simulink model "Demo_FrictionSensor_cs"  (Simulink 7.6)
settings: Solver=ode5  SolverMode=SingleTasking  StartTime=0.0  StopTime=12  FixedStep=1/200  RelTol=1e-3
PreLoadFcn:
  | check_NUTS_defined;
  | 
  | assignin('base',['model_closed_' bdroot],false);
InitFcn:
  | PreScanExperimentInitFcn(bdroot)
StopFcn:
  | PreScanExperimentStopFcn(bdroot)
undefined symbols (not defined in the file): DiscIntNeverNeededParam, warningInitialVelocity, x0, x_ini_VRML, y_ini_VRML, z_ini_VRML
libraries: simulink x40, PreScanSimulinkLibrary x15, simulink_extras x9, PreScanUsefulBlocks x3
(part 6 of 7)

== system Demo_FrictionSensor_cs/Audi_A8_1/PathFollower_Preview_1/LateralController/SteeringWheelAngle/FirstOrderDynamics ==
  In : Inport
  TimeConstant[s] : Inport  Port=2
  Reset : Inport  Port=3
  x0 : Inport  Port=4
  1|TimeConstant : Product  Inputs=*/  SaturateOnIntegerOverflow=on  InputSameDT=on  OutDataTypeStr=Inherit: Same as first input
  Discrete-Time Integrator : DiscreteIntegrator  ExternalReset=rising  InitialConditionSource=external  InitialCondition=x0  SampleTime=CSSampleTime  ICPrevOutput=DiscIntNeverNeededParam  ICPrevScaledInput=DiscIntNeverNeededParam
  IC : InitialCondition  Value=0
  Saturation : Saturate  UpperLimit=1e300  LowerLimit=0.001
  Sum : Sum  Inputs=-+|  SaturateOnIntegerOverflow=on  InputSameDT=on  OutDataTypeStr=Inherit: Same as first input
  Out : Outport
  wires:
  IC/1 -> Discrete-Time Integrator/3
  In/1 -> Sum/2
  x0/1 -> IC/1
  Reset/1 -> Discrete-Time Integrator/2
  1|TimeConstant/1 -> Discrete-Time Integrator/1
  Sum/1 -> 1|TimeConstant/1
  Saturation/1 -> 1|TimeConstant/2
  TimeConstant[s]/1 -> Saturation/1
  Discrete-Time Integrator/1 -> Out/1, Sum/1

== system Demo_FrictionSensor_cs/Audi_A8_1/PathFollower_Preview_1/LateralController/SteeringWheelAngle/Sat_Total ==
  In : Inport
  Sat_Limit : Inport  Port=2
  Gain1 : Gain  Gain=-1  SaturateOnIntegerOverflow=on  OutDataTypeStr=Inherit: Same as input  ParamDataTypeStr=Inherit: Same as input
  RelOp_UL : RelationalOperator
  RelOp_UL1 : RelationalOperator  Operator=<=
  Sum : Sum  Inputs=++|  SaturateOnIntegerOverflow=on
  Switch : Switch  Threshold=0.5  SaturateOnIntegerOverflow=on
  Switch1 : Switch  Threshold=0.5  SaturateOnIntegerOverflow=on
  Sat_Total : Outport
  Sat_Info : Outport  Port=2
  wires:
  Sat_Limit/1 -> Gain1/1, Switch/1, RelOp_UL/2
  RelOp_UL/1 -> Switch/2, Sum/2
  Switch/1 -> RelOp_UL1/1, Switch1/3
  Gain1/1 -> RelOp_UL1/2, Switch1/1
  RelOp_UL1/1 -> Switch1/2, Sum/1
  In/1 -> Switch/3, RelOp_UL/1
  Switch1/1 -> Sat_Total/1
  Sum/1 -> Sat_Info/1

== system Demo_FrictionSensor_cs/Audi_A8_1/PathFollower_Preview_1/LongitudinalController/If Desired Velocity ~= 0/PID Controller ==
  e : Inport
  Derivative Gain : Gain  Gain=D  SaturateOnIntegerOverflow=on  OutDataTypeStr=Inherit: Same as input  ParamDataTypeStr=Inherit: Same as input
  Discrete-Time Integrator : DiscreteIntegrator  gainval=1  SampleTime=CSSampleTime  ICPrevOutput=DiscIntNeverNeededParam  ICPrevScaledInput=DiscIntNeverNeededParam
  Filter : DiscreteIntegrator  gainval=1  SampleTime=CSSampleTime  ICPrevOutput=DiscIntNeverNeededParam  ICPrevScaledInput=DiscIntNeverNeededParam
  Integral Gain : Gain  Gain=I  SaturateOnIntegerOverflow=on  OutDataTypeStr=Inherit: Same as input  ParamDataTypeStr=Inherit: Same as input
  Proportional Gain : Gain  Gain=P  SaturateOnIntegerOverflow=on  OutDataTypeStr=Inherit: Same as input  ParamDataTypeStr=Inherit: Same as input
  Sum : Sum  Inputs=+++  SaturateOnIntegerOverflow=on  InputSameDT=on  OutDataTypeStr=Inherit: Same as first input
  Sum1 : Sum  Inputs=|+-  SaturateOnIntegerOverflow=on  InputSameDT=on  OutDataTypeStr=Inherit: Same as first input
  u : Outport  InitialOutput=0
  wires:
  Sum1/1 -> Filter/1, Sum/3
  Filter/1 -> Sum1/2
  Derivative Gain/1 -> Sum1/1
  Sum/1 -> u/1
  e/1 -> Integral Gain/1, Proportional Gain/1, Derivative Gain/1
  Discrete-Time Integrator/1 -> Sum/2
  Proportional Gain/1 -> Sum/1
  Integral Gain/1 -> Discrete-Time Integrator/1

== system Demo_FrictionSensor_cs/Audi_A8_1/PreScan_Contact_Sensor/Vehicle Local to World/state2FullState/Transformation_BODY2GLOBAL1 ==
  POSvector_BODY_[m] : Inport
  angles_BODYwrtGLOB_[rad] : Inport  Port=2
  Dot Product : DotProduct  InputSameDT=on  OutDataTypeStr=Inherit: Inherit via internal rule
  Dot Product1 : DotProduct  InputSameDT=on  OutDataTypeStr=Inherit: Inherit via internal rule
  Dot Product2 : DotProduct  InputSameDT=on  OutDataTypeStr=Inherit: Inherit via internal rule
  Fcn10 : Fcn  Expr=cos(u(1))*sin(u(2))*sin(u(3))-sin(u(1))*cos(u(3))
  Fcn11 : Fcn  Expr=cos(u(1))*sin(u(2))*cos(u(3))+sin(u(1))*sin(u(3))
  Fcn12 : Fcn  Expr=sin(u(1))*cos(u(2))
  Fcn13 : Fcn  Expr=sin(u(1))*sin(u(2))*sin(u(3))+cos(u(1))*cos(u(3))
  Fcn14 : Fcn  Expr=sin(u(1))*sin(u(2))*cos(u(3))-cos(u(1))*sin(u(3))
  Fcn15 : Fcn  Expr=-sin(u(2))
  Fcn16 : Fcn  Expr=cos(u(2))*sin(u(3))
  Fcn17 : Fcn  Expr=cos(u(2))*cos(u(3))
  Fcn9 : Fcn  Expr=cos(u(1))*cos(u(2))
  Mux1 : Mux  Inputs=9
  Mux3 : Mux  Inputs=3
  Selector : Selector  InputPortWidth=9  IndexOptions=Index vector (dialog)  Indices=[1 2 3]  OutputSizes=1
  Selector1 : Selector  InputPortWidth=9  IndexOptions=Index vector (dialog)  Indices=[4 5 6]  OutputSizes=1
  Selector2 : Selector  InputPortWidth=9  IndexOptions=Index vector (dialog)  Indices=[7 8 9]  OutputSizes=1
  rot_xyz 2 rot_zyx : Selector  InputPortWidth=3  IndexOptions=Index vector (dialog)  Indices=[3 2 1]  OutputSizes=1
  POSvector_GLOBAL_[m] : Outport
  wires:
  angles_BODYwrtGLOB_[rad]/1 -> rot_xyz 2 rot_zyx/1
  Mux3/1 -> POSvector_GLOBAL_[m]/1
  rot_xyz 2 rot_zyx/1 -> Fcn17/1, Fcn16/1, Fcn15/1, Fcn14/1, Fcn13/1, Fcn12/1, Fcn11/1, Fcn10/1, Fcn9/1
  Dot Product1/1 -> Mux3/2
  Dot Product2/1 -> Mux3/3
  Selector2/1 -> Dot Product2/2
  Selector1/1 -> Dot Product1/2
  Dot Product/1 -> Mux3/1
  POSvector_BODY_[m]/1 -> Dot Product/1, Dot Product1/1, Dot Product2/1
  Selector/1 -> Dot Product/2
  Mux1/1 -> Selector2/1, Selector1/1, Selector/1  "RotationMatrix"
  Fcn17/1 -> Mux1/9
  Fcn16/1 -> Mux1/8
  Fcn15/1 -> Mux1/7
  Fcn14/1 -> Mux1/6
  Fcn13/1 -> Mux1/5
  Fcn12/1 -> Mux1/4
  Fcn11/1 -> Mux1/3
  Fcn10/1 -> Mux1/2
  Fcn9/1 -> Mux1/1

== system Demo_FrictionSensor_cs/Audi_A8_1/PreScan_Contact_Sensor/Vehicle Local to World/state2FullState/limit roll ==
  RPY : Inport
  Demux : Demux  Outputs=3
  Mux1 : Mux  Inputs=3
  Substitute 90 & 270 deg (and its plurals) : Subsystem
  RPYcor : Outport
  wires:
  Demux/1 -> Substitute 90 & 270 deg (and its plurals)/1(Angle [rad])
  Demux/2 -> Mux1/2
  Demux/3 -> Mux1/3
  RPY/1 -> Demux/1
  Mux1/1 -> RPYcor/1
  Substitute 90 & 270 deg (and its plurals)/1(Subst Angle [rad]) -> Mux1/1

== system Demo_FrictionSensor_cs/Audi_A8_1/PreScan_Contact_Sensor/Wheels Local to World/conv_RotWheelFL/RotMat2AxisAngle ==
  RotMat_Visu : Inport
  Data Type Conversion : DataTypeConversion
  Divide : Product  Inputs=*/
  Gain : Gain  Gain=2
  Mux : Mux  Inputs=3
  Mux1 : Mux  Inputs=2
  Saturation1 : Saturate  UpperLimit=3-0.001  LowerLimit=-1+0.001
  Trigonometric Function : Trigonometry
  U1 : Fcn  Expr=u[6]-u[8]
  U2 : Fcn  Expr=u[7]-u[3]
  U3 : Fcn  Expr=u[2]-u[4]
  U_Phi : Fcn  Expr=u[1]+u[5]+u[9]
  U_Phi1 : Fcn  Expr=acos((u(1)-1)/2)
  U_Phi2 : Fcn  Expr=acos((u(1)-1)/2)
  Angles_Visu : Outport
  wires:
  Data Type Conversion/1 -> Mux1/2
  RotMat_Visu/1 -> U1/1, U2/1, U3/1, U_Phi/1
  Trigonometric Function/1 -> Gain/1
  U1/1 -> Mux/1
  U2/1 -> Mux/2
  U3/1 -> Mux/3
  Mux/1 -> Divide/1
  Gain/1 -> Divide/2
  Mux1/1 -> Angles_Visu/1
  Divide/1 -> Mux1/1
  U_Phi/1 -> U_Phi1/1, Saturation1/1
  U_Phi1/1 -> Data Type Conversion/1
  Saturation1/1 -> U_Phi2/1
  U_Phi2/1 -> Trigonometric Function/1

== system Demo_FrictionSensor_cs/Audi_A8_1/PreScan_Contact_Sensor/Wheels Local to World/conv_RotWheelFR/RotMat2AxisAngle ==
  RotMat_Visu : Inport
  Data Type Conversion : DataTypeConversion
  Divide : Product  Inputs=*/
  Gain : Gain  Gain=2
  Mux : Mux  Inputs=3
  Mux1 : Mux  Inputs=2
  Saturation1 : Saturate  UpperLimit=3-0.001  LowerLimit=-1+0.001
  Trigonometric Function : Trigonometry
  U1 : Fcn  Expr=u[6]-u[8]
  U2 : Fcn  Expr=u[7]-u[3]
  U3 : Fcn  Expr=u[2]-u[4]
  U_Phi : Fcn  Expr=u[1]+u[5]+u[9]
  U_Phi1 : Fcn  Expr=acos((u(1)-1)/2)
  U_Phi2 : Fcn  Expr=acos((u(1)-1)/2)
  Angles_Visu : Outport
  wires:
  U_Phi2/1 -> Trigonometric Function/1
  Saturation1/1 -> U_Phi2/1
  U_Phi1/1 -> Data Type Conversion/1
  U_Phi/1 -> Saturation1/1, U_Phi1/1
  Divide/1 -> Mux1/1
  Mux1/1 -> Angles_Visu/1
  Gain/1 -> Divide/2
  Mux/1 -> Divide/1
  U3/1 -> Mux/3
  U2/1 -> Mux/2
  U1/1 -> Mux/1
  Trigonometric Function/1 -> Gain/1
  RotMat_Visu/1 -> U_Phi/1, U3/1, U2/1, U1/1
  Data Type Conversion/1 -> Mux1/2

== system Demo_FrictionSensor_cs/Audi_A8_1/PreScan_Contact_Sensor/Wheels Local to World/conv_RotWheelRL/RotMat2AxisAngle ==
  RotMat_Visu : Inport
  Data Type Conversion : DataTypeConversion
  Divide : Product  Inputs=*/
  Gain : Gain  Gain=2
  Mux : Mux  Inputs=3
  Mux1 : Mux  Inputs=2
  Saturation1 : Saturate  UpperLimit=3-0.001  LowerLimit=-1+0.001
  Trigonometric Function : Trigonometry
  U1 : Fcn  Expr=u[6]-u[8]
  U2 : Fcn  Expr=u[7]-u[3]
  U3 : Fcn  Expr=u[2]-u[4]
  U_Phi : Fcn  Expr=u[1]+u[5]+u[9]
  U_Phi1 : Fcn  Expr=acos((u(1)-1)/2)
  U_Phi2 : Fcn  Expr=acos((u(1)-1)/2)
  Angles_Visu : Outport
  wires:
  U_Phi2/1 -> Trigonometric Function/1
  Saturation1/1 -> U_Phi2/1
  U_Phi1/1 -> Data Type Conversion/1
  U_Phi/1 -> Saturation1/1, U_Phi1/1
  Divide/1 -> Mux1/1
  Mux1/1 -> Angles_Visu/1
  Gain/1 -> Divide/2
  Mux/1 -> Divide/1
  U3/1 -> Mux/3
  U2/1 -> Mux/2
  U1/1 -> Mux/1
  Trigonometric Function/1 -> Gain/1
  RotMat_Visu/1 -> U_Phi/1, U3/1, U2/1, U1/1
  Data Type Conversion/1 -> Mux1/2

== system Demo_FrictionSensor_cs/Audi_A8_1/PreScan_Contact_Sensor/Wheels Local to World/conv_RotWheelRR/RotMat2AxisAngle ==
  RotMat_Visu : Inport
  Data Type Conversion : DataTypeConversion
  Divide : Product  Inputs=*/
  Gain : Gain  Gain=2
  Mux : Mux  Inputs=3
  Mux1 : Mux  Inputs=2
  Saturation1 : Saturate  UpperLimit=3-0.001  LowerLimit=-1+0.001
  Trigonometric Function : Trigonometry
  U1 : Fcn  Expr=u[6]-u[8]
  U2 : Fcn  Expr=u[7]-u[3]
  U3 : Fcn  Expr=u[2]-u[4]
  U_Phi : Fcn  Expr=u[1]+u[5]+u[9]
  U_Phi1 : Fcn  Expr=acos((u(1)-1)/2)
  U_Phi2 : Fcn  Expr=acos((u(1)-1)/2)
  Angles_Visu : Outport
  wires:
  U_Phi2/1 -> Trigonometric Function/1
  Saturation1/1 -> U_Phi2/1
  U_Phi1/1 -> Data Type Conversion/1
  U_Phi/1 -> Saturation1/1, U_Phi1/1
  Divide/1 -> Mux1/1
  Mux1/1 -> Angles_Visu/1
  Gain/1 -> Divide/2
  Mux/1 -> Divide/1
  U3/1 -> Mux/3
  U2/1 -> Mux/2
  U1/1 -> Mux/1
  Trigonometric Function/1 -> Gain/1
  RotMat_Visu/1 -> U_Phi/1, U3/1, U2/1, U1/1
  Data Type Conversion/1 -> Mux1/2

== system Demo_FrictionSensor_cs/Audi_A8_1/PreScan_Contact_Sensor/Wheels Local to World/conv_TransWheelFL/pos_ini_Visu ==
  Constant : Constant  Value=x_ini_VRML
  Constant1 : Constant  Value=y_ini_VRML
  Constant2 : Constant  Value=z_ini_VRML
  Mux1 : Mux  Inputs=3
  pos_ini_Visu : Outport
  wires:
  Constant/1 -> Mux1/1
  Mux1/1 -> pos_ini_Visu/1
  Constant1/1 -> Mux1/2
  Constant2/1 -> Mux1/3

== system Demo_FrictionSensor_cs/Audi_A8_1/PreScan_Contact_Sensor/Wheels Local to World/conv_TransWheelFL/transISO2Visu ==
  transISO : Inport
  Demux : Demux  Outputs=3
  trans_x_Visu : Outport
  trans_y_Visu : Outport  Port=2
  trans_z_Visu : Outport  Port=3
  wires:
  Demux/2 -> trans_y_Visu/1  "rot_y"
  Demux/1 -> trans_x_Visu/1
  transISO/1 -> Demux/1
  Demux/3 -> trans_z_Visu/1

== system Demo_FrictionSensor_cs/Audi_A8_1/PreScan_Contact_Sensor/Wheels Local to World/conv_TransWheelFR/pos_ini_Visu ==
  Constant : Constant  Value=x_ini_VRML
  Constant1 : Constant  Value=y_ini_VRML
  Constant2 : Constant  Value=z_ini_VRML
  Mux1 : Mux  Inputs=3
  pos_ini_Visu : Outport
  wires:
  Constant2/1 -> Mux1/3
  Constant1/1 -> Mux1/2
  Mux1/1 -> pos_ini_Visu/1
  Constant/1 -> Mux1/1

== system Demo_FrictionSensor_cs/Audi_A8_1/PreScan_Contact_Sensor/Wheels Local to World/conv_TransWheelFR/transISO2Visu ==
  transISO : Inport
  Demux : Demux  Outputs=3
  trans_x_Visu : Outport
  trans_y_Visu : Outport  Port=2
  trans_z_Visu : Outport  Port=3
  wires:
  Demux/2 -> trans_y_Visu/1  "rot_y"
  Demux/1 -> trans_x_Visu/1
  transISO/1 -> Demux/1
  Demux/3 -> trans_z_Visu/1

== system Demo_FrictionSensor_cs/Audi_A8_1/PreScan_Contact_Sensor/Wheels Local to World/conv_TransWheelRL/pos_ini_Visu ==
  Constant : Constant  Value=x_ini_VRML
  Constant1 : Constant  Value=y_ini_VRML
  Constant2 : Constant  Value=z_ini_VRML
  Mux1 : Mux  Inputs=3
  pos_ini_Visu : Outport
  wires:
  Constant2/1 -> Mux1/3
  Constant1/1 -> Mux1/2
  Mux1/1 -> pos_ini_Visu/1
  Constant/1 -> Mux1/1

== system Demo_FrictionSensor_cs/Audi_A8_1/PreScan_Contact_Sensor/Wheels Local to World/conv_TransWheelRL/transISO2Visu ==
  transISO : Inport
  Demux : Demux  Outputs=3
  trans_x_Visu : Outport
  trans_y_Visu : Outport  Port=2
  trans_z_Visu : Outport  Port=3
  wires:
  Demux/2 -> trans_y_Visu/1  "rot_y"
  Demux/1 -> trans_x_Visu/1
  transISO/1 -> Demux/1
  Demux/3 -> trans_z_Visu/1

== system Demo_FrictionSensor_cs/Audi_A8_1/PreScan_Contact_Sensor/Wheels Local to World/conv_TransWheelRR/pos_ini_Visu ==
  Constant : Constant  Value=x_ini_VRML
  Constant1 : Constant  Value=y_ini_VRML
  Constant2 : Constant  Value=z_ini_VRML
  Mux1 : Mux  Inputs=3
  pos_ini_Visu : Outport
  wires:
  Constant2/1 -> Mux1/3
  Constant1/1 -> Mux1/2
  Mux1/1 -> pos_ini_Visu/1
  Constant/1 -> Mux1/1

== system Demo_FrictionSensor_cs/Audi_A8_1/PreScan_Contact_Sensor/Wheels Local to World/conv_TransWheelRR/transISO2Visu ==
  transISO : Inport
  Demux : Demux  Outputs=3
  trans_x_Visu : Outport
  trans_y_Visu : Outport  Port=2
  trans_z_Visu : Outport  Port=3
  wires:
  Demux/2 -> trans_y_Visu/1  "rot_y"
  Demux/1 -> trans_x_Visu/1
  transISO/1 -> Demux/1
  Demux/3 -> trans_z_Visu/1

== system Demo_FrictionSensor_cs/Audi_A8_1/Trajectories/Traj2State1/Traj2State2/MuxState ==
  x [m] : Inport
  y [m] : Inport  Port=2
  z [m] : Inport  Port=3
  dx [m/s] : Inport  Port=4
  dy [m/s] : Inport  Port=5
  dz [m/s] : Inport  Port=6
  R [rad] : Inport  Port=7
  P [rad] : Inport  Port=8
  Y [rad] : Inport  Port=9
  Mux : Mux  Inputs=9
  state : Outport
  wires:
  z [m]/1 -> Mux/3
  y [m]/1 -> Mux/2
  x [m]/1 -> Mux/1
  Y [rad]/1 -> Mux/9
  P [rad]/1 -> Mux/8
  R [rad]/1 -> Mux/7
  dz [m/s]/1 -> Mux/6
  dy [m/s]/1 -> Mux/5
  dx [m/s]/1 -> Mux/4
  Mux/1 -> state/1

== system Demo_FrictionSensor_cs/Audi_A8_1/Trajectories/Traj2State1/Traj2State2/Traj2MuxState_Ext ==
  Traj : Inport
  Terminator{1..9} (9 alike) : Terminator
  demux : Subsystem
  x [m] : Outport
  y [m] : Outport  Port=2
  z [m] : Outport  Port=3
  dx [m/s] : Outport  Port=4
  dy [m/s] : Outport  Port=5
  dz [m/s] : Outport  Port=6
  R [rad] : Outport  Port=7
  P [rad] : Outport  Port=8
  Y [rad] : Outport  Port=9
  wires:
  demux/9(Y) -> Y [rad]/1
  demux/7(R) -> R [rad]/1
  demux/5(vely) -> dy [m/s]/1
  demux/4(velx) -> dx [m/s]/1
  demux/10(velR) -> Terminator4/1
  demux/11(velP) -> Terminator5/1
  demux/12(velY) -> Terminator1/1
  demux/13(accx) -> Terminator8/1
  demux/14(accy) -> Terminator9/1
  demux/15(accz) -> Terminator7/1
  demux/18(accY) -> Terminator2/1
  demux/16(accR) -> Terminator3/1
  demux/17(accP) -> Terminator6/1
  demux/3(z) -> z [m]/1
  Traj/1 -> demux/1(traj)
  demux/6(velz) -> dz [m/s]/1
  demux/1(x) -> x [m]/1
  demux/2(y) -> y [m]/1
  demux/8(P) -> P [rad]/1

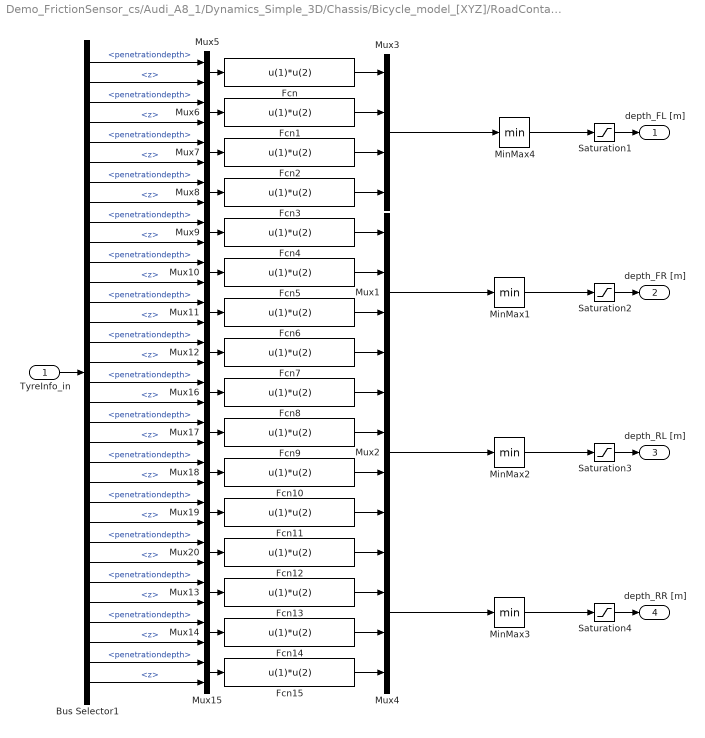
== system Demo_FrictionSensor_cs/Audi_A8_1/Dynamics_Simple_3D/Chassis/Bicycle_model_[XYZ]/RoadContact/Penetration depth ==
  TyreInfo_in : Inport
  Bus Selector1 : BusSelector  OutputSignals=TireFL.cp0.penetrationdepth,TireFL.cp0.normal.z,TireFL.cp1.penetrationdepth,TireFL.cp1.normal.z,TireFL.cp2.penetrationdepth,TireFL.cp2.normal.z,TireFL.cp3.penetrationdepth,TireFL.cp3.normal.z,TireFR.cp0.penetrationdepth,TireFR.cp0.normal.z,TireFR.cp1.penetrationdepth,TireFR.cp1.normal.z,TireFR.cp2.penetrationdepth,TireFR.cp2.normal.z,TireFR.cp3.penetrationdepth,TireFR.cp3.normal.z,TireRL.cp0.penetrationdepth,TireRL.cp0.normal.z,TireRL.cp1.penetrationdepth,TireRL.cp1.normal.z,TireRL.cp2.penetrationdepth,TireRL.cp2.normal.z,TireRL.cp3.penetrationdepth,TireRL.cp3.normal.z,TireRR.cp0.penetrationdepth,TireRR.cp0.normal.z,TireRR.cp1.penetrationdepth,TireRR.cp1.normal.z,TireRR.cp2.penetrationdepth,TireRR.cp2.normal.z,TireRR.cp3.penetrationdepth,TireRR.cp3.normal.z
  Fcn{,1..15} (16 alike) : Fcn  Expr=u(1)*u(2)
  MinMax{1..4} (4 alike) : MinMax
  Mux{1..4} (4 alike) : Mux
  Mux{5..20} (16 alike) : Mux  Inputs=2
  Saturation{1..4} (4 alike) : Saturate  UpperLimit=0  LowerLimit=-inf
  depth_FL [m] : Outport
  depth_FR [m] : Outport  Port=2
  depth_RL [m] : Outport  Port=3
  depth_RR [m] : Outport  Port=4
  wires:
  Saturation4/1 -> depth_RR [m]/1
  Saturation3/1 -> depth_RL [m]/1
  TyreInfo_in/1 -> Bus Selector1/1
  Saturation2/1 -> depth_FR [m]/1
  Saturation1/1 -> depth_FL [m]/1
  Mux3/1 -> MinMax4/1
  MinMax3/1 -> Saturation4/1
  Mux4/1 -> MinMax3/1
  Bus Selector1/1 -> Mux5/1  "<penetrationdepth>"
  Bus Selector1/2 -> Mux5/2  "<z>"
  Bus Selector1/3 -> Mux6/1  "<penetrationdepth>"
  Bus Selector1/4 -> Mux6/2  "<z>"
  Bus Selector1/5 -> Mux7/1  "<penetrationdepth>"
  Bus Selector1/6 -> Mux7/2  "<z>"
  Bus Selector1/7 -> Mux8/1  "<penetrationdepth>"
  Bus Selector1/8 -> Mux8/2  "<z>"
  Bus Selector1/9 -> Mux9/1  "<penetrationdepth>"
  Bus Selector1/10 -> Mux9/2  "<z>"
  Bus Selector1/11 -> Mux10/1  "<penetrationdepth>"
  Bus Selector1/12 -> Mux10/2  "<z>"
  Bus Selector1/13 -> Mux11/1  "<penetrationdepth>"
  Bus Selector1/14 -> Mux11/2  "<z>"
  Bus Selector1/15 -> Mux12/1  "<penetrationdepth>"
  Bus Selector1/16 -> Mux12/2  "<z>"
  Bus Selector1/17 -> Mux16/1  "<penetrationdepth>"
  Bus Selector1/18 -> Mux16/2  "<z>"
  Bus Selector1/19 -> Mux17/1  "<penetrationdepth>"
  Bus Selector1/20 -> Mux17/2  "<z>"
  Bus Selector1/21 -> Mux18/1  "<penetrationdepth>"
  Bus Selector1/22 -> Mux18/2  "<z>"
  Bus Selector1/23 -> Mux19/1  "<penetrationdepth>"
  Bus Selector1/24 -> Mux19/2  "<z>"
  Bus Selector1/25 -> Mux20/1  "<penetrationdepth>"
  Bus Selector1/26 -> Mux20/2  "<z>"
  Bus Selector1/27 -> Mux13/1  "<penetrationdepth>"
  Bus Selector1/28 -> Mux13/2  "<z>"
  Bus Selector1/29 -> Mux14/1  "<penetrationdepth>"
  Bus Selector1/30 -> Mux14/2  "<z>"
  Bus Selector1/31 -> Mux15/1  "<penetrationdepth>"
  Bus Selector1/32 -> Mux15/2  "<z>"
  MinMax4/1 -> Saturation1/1
  Mux2/1 -> MinMax2/1
  MinMax2/1 -> Saturation3/1
  Mux1/1 -> MinMax1/1
  MinMax1/1 -> Saturation2/1
  Mux5/1 -> Fcn/1
  Mux6/1 -> Fcn1/1
  Mux7/1 -> Fcn2/1
  Mux8/1 -> Fcn3/1
  Mux9/1 -> Fcn4/1
  Mux10/1 -> Fcn5/1
  Mux11/1 -> Fcn6/1
  Mux12/1 -> Fcn7/1
  Fcn/1 -> Mux3/1
  Fcn1/1 -> Mux3/2
  Fcn2/1 -> Mux3/3
  Fcn3/1 -> Mux3/4
  Fcn4/1 -> Mux1/1
  Fcn5/1 -> Mux1/2
  Fcn6/1 -> Mux1/3
  Fcn7/1 -> Mux1/4
  Mux16/1 -> Fcn8/1
  Mux17/1 -> Fcn9/1
  Mux18/1 -> Fcn10/1
  Mux19/1 -> Fcn11/1
  Mux20/1 -> Fcn12/1
  Mux13/1 -> Fcn13/1
  Mux14/1 -> Fcn14/1
  Mux15/1 -> Fcn15/1
  Fcn8/1 -> Mux2/1
  Fcn9/1 -> Mux2/2
  Fcn10/1 -> Mux2/3
  Fcn11/1 -> Mux2/4
  Fcn12/1 -> Mux4/1
  Fcn13/1 -> Mux4/2
  Fcn14/1 -> Mux4/3
  Fcn15/1 -> Mux4/4

== system Demo_FrictionSensor_cs/Audi_A8_1/Dynamics_Simple_3D/Chassis/Bicycle_model_[XYZ]/RoadContact/RoadGeometry ==
  TyreInfo_in : Inport
  Calc_banking : Subsystem
  Calc_slope : Subsystem
  Calc_z : Subsystem
  DocBlock : simulink/Model-Wide Utilities/DocBlock  SystemSampleTime=-1  DocumentType=Text
      content=|
      | This block determines, based on the z-coordinates of the road in
      | correspondence of the contact points,
      | - the z-coordinate of the road in correspondence of the middle point of the
      |   vehicle (z);
      | - the slope angle of the road (alpha, positive when downhill);
      | - the banking angle of the road (beta, positive when counter-clockwise when
      |   looking from the front of the vehicle).
      |
      | For every wheel there are 4 contact points (cp0, cp1, cp2, cp3) defined in
      | TyreInfo_in. Not all 4 contact points reports always a value, depending on
      | different conditions there might be contact points that do not report a
      | value. These points report in this case to 0. If the tyre is lifted from
      | the road, all contact points report 0. Because of this reason, the
      | value of the contact point that reports the largest negative value of the
      | penetration depth is used. If all values of the penetration depth are 0,
      | then a maximum gradient is applied to avoid jumps to 0 in the z signal.
      | The maximum gradient is fixed to -6 [m/s^2], this value is large enough for
      | a vehicle driving at 30 [m/s] downhill on a gradient of 20 [%]. Further, a
      | first order low pass linear filter with a bandwidth of 1 [Hz] is applied.
      | This filter removes high frequencies components in the signal, when one
      | wheel is lifted (e.g. drive in a corner with a large lateral acceleration).
      | The bandwidth of 1 [Hz] is large enough to include the main frequencies
      | that occurr in the vehicle roll, pitch and vertical movements.
      |
      | z, slope and banking are determined as follows:
      |
      | z        = (+ zFL + zFR + zRL + zRR) / 4            (Calc_z)
      | slope    = (- zFL - zFR + zRL + zRR) / (2*p.l)      (Calc_slope)
      | banking  = (+ zFL - zFR + zRL - zRR) / (2*p.width)  (Calc_banking)
  Mux4 : Mux
  zFL_lowerpenetrationdetph : Subsystem
  zFL_tyreinfo : Subsystem
  zFR_lowerpenetrationdetph : Subsystem
  zFR_tyreinfo : Subsystem
  zRL_lowerpenetrationdetph : Subsystem
  zRL_tyreinfo : Subsystem
  zRR_lowerpenetrationdetph : Subsystem
  zRR_tyreinfo : Subsystem
  z : Outport
  slope : Outport  Port=2
  banking : Outport  Port=3
  wires:
  zRR_tyreinfo/3(normal_z) -> zRR_lowerpenetrationdetph/3(normal_z)
  zRR_tyreinfo/2(position_z) -> zRR_lowerpenetrationdetph/2(position_z)
  zRR_tyreinfo/1(penetrationdepth) -> zRR_lowerpenetrationdetph/1(penetrationdepth)
  zRL_tyreinfo/3(normal_z) -> zRL_lowerpenetrationdetph/3(normal_z)
  zRL_tyreinfo/2(position_z) -> zRL_lowerpenetrationdetph/2(position_z)
  zRL_tyreinfo/1(penetrationdepth) -> zRL_lowerpenetrationdetph/1(penetrationdepth)
  zFR_tyreinfo/3(normal_z) -> zFR_lowerpenetrationdetph/3(normal_z)
  zFR_tyreinfo/2(position_z) -> zFR_lowerpenetrationdetph/2(position_z)
  zFR_tyreinfo/1(penetrationdepth) -> zFR_lowerpenetrationdetph/1(penetrationdepth)
  zFL_tyreinfo/3(normal_z) -> zFL_lowerpenetrationdetph/3(normal_z)
  zFL_tyreinfo/2(position_z) -> zFL_lowerpenetrationdetph/2(position_z)
  zFL_tyreinfo/1(penetrationdepth) -> zFL_lowerpenetrationdetph/1(penetrationdepth)
  zRR_lowerpenetrationdetph/1(z) -> Mux4/4
  zRL_lowerpenetrationdetph/1(z) -> Mux4/3
  zFR_lowerpenetrationdetph/1(z) -> Mux4/2
  zFL_lowerpenetrationdetph/1(z) -> Mux4/1
  Calc_banking/1(banking) -> banking/1
  Calc_slope/1(slope) -> slope/1
  Mux4/1 -> Calc_banking/1(zi), Calc_slope/1(zi), Calc_z/1(zi)
  Calc_z/1(z) -> z/1
  TyreInfo_in/1 -> zRR_tyreinfo/1(In1), zRL_tyreinfo/1(In1), zFR_tyreinfo/1(In1), zFL_tyreinfo/1(In1)

== system Demo_FrictionSensor_cs/Audi_A8_1/Dynamics_Simple_3D/Chassis/Bicycle_model_[XYZ]/X_Motion/Air&RoadResistance ==
  vx_[ms-1] : Inport
  slope_[rad] : Inport  Port=2
  Gain : Gain  Gain=1/p.Rw
  Mux4 : Mux  Inputs=2
  Road & Aerodyn Resistances : Fcn  Expr=p.Rroad*cos(u(2)) + p.Rair*u(1)^2
  Saturation1 : Saturate  UpperLimit=5/15  LowerLimit=-5/15
  Sign : Signum
  "[ms-1] 2 [rads-1]" : Gain  Gain=1/p.Rw  SaturateOnIntegerOverflow=on  OutDataTypeStr=Inherit: Same as input  ParamDataTypeStr=Inherit: Same as input
  signed load1 : Product  SaturateOnIntegerOverflow=on  InputSameDT=on  OutDataTypeStr=Inherit: Same as first input
  Resistance_Force : Outport
  wires:
  signed load1/1 -> Resistance_Force/1  "F_[N]"
  vx_[ms-1]/1 -> "[ms-1] 2 [rads-1]"/1, Mux4/1
  Saturation1/1 -> Sign/1
  "[ms-1] 2 [rads-1]"/1 -> Saturation1/1
  Sign/1 -> signed load1/2  "sign"
  Road & Aerodyn Resistances/1 -> Gain/1  "ResistanceTorque_[Nm]"
  Mux4/1 -> Road & Aerodyn Resistances/1
  slope_[rad]/1 -> Mux4/2
  Gain/1 -> signed load1/1  "ResistanceForce_[N]"

== system Demo_FrictionSensor_cs/Audi_A8_1/Dynamics_Simple_3D/Chassis/Bicycle_model_[XYZ]/X_Motion/BrakeSystem ==
  vx_[ms-1] : Inport
  BrakePressure_[bar] : Inport  Port=2
  Gain : Gain  Gain=1/p.Rw
  Saturation : Saturate  UpperLimit=p.PBrakeMax  LowerLimit=0
  Saturation1 : Saturate  UpperLimit=5/15  LowerLimit=-5/15
  Sign : Signum
  "[ms-1] 2 [rads-1]" : Gain  Gain=1/p.Rw  SaturateOnIntegerOverflow=on  OutDataTypeStr=Inherit: Same as input  ParamDataTypeStr=Inherit: Same as input
  braking Q factor : Gain  Gain=p.Qfac  SaturateOnIntegerOverflow=on  OutDataTypeStr=Inherit: Same as input  ParamDataTypeStr=Inherit: Same as input
  signed load1 : Product  SaturateOnIntegerOverflow=on  InputSameDT=on  OutDataTypeStr=Inherit: Same as first input
  BrakeForce : Outport
  BrakeTorqueAbs : Outport  Port=2
  wires:
  braking Q factor/1 -> BrakeTorqueAbs/1, Gain/1
  BrakePressure_[bar]/1 -> Saturation/1
  Saturation/1 -> braking Q factor/1
  vx_[ms-1]/1 -> "[ms-1] 2 [rads-1]"/1
  Saturation1/1 -> Sign/1
  "[ms-1] 2 [rads-1]"/1 -> Saturation1/1
  Sign/1 -> signed load1/2  "sign"
  signed load1/1 -> BrakeForce/1
  Gain/1 -> signed load1/1

== system Demo_FrictionSensor_cs/Audi_A8_1/Dynamics_Simple_3D/Chassis/Bicycle_model_[XYZ]/X_Motion/Configurable Subsystem ==
  In1 : Inport
  In2 : Inport  Port=2
  In3 : Inport  Port=3
  Discrete-Time Integrator : DiscreteIntegrator  ExternalReset=level  InitialConditionSource=external  SampleTime=TimeStep  ICPrevOutput=DiscIntNeverNeededParam  ICPrevScaledInput=DiscIntNeverNeededParam
  Out1 : Outport
  wires:
  Discrete-Time Integrator/1 -> Out1/1
  In3/1 -> Discrete-Time Integrator/3
  In2/1 -> Discrete-Time Integrator/2
  In1/1 -> Discrete-Time Integrator/1

== system Demo_FrictionSensor_cs/Audi_A8_1/Dynamics_Simple_3D/Chassis/Bicycle_model_[XYZ]/X_Motion/Configurable Subsystem1 ==
  In1 : Inport
  Discrete Torsional damping : DiscreteTransferFcn  Numerator="[  1-exp(-( (TimeStep) / 0.1) )  ]"  Denominator="[  1   -exp(-( (TimeStep) / 0.1) )   ]"  SampleTime=TimeStep
  Out1 : Outport
  wires:
  Discrete Torsional damping/1 -> Out1/1
  In1/1 -> Discrete Torsional damping/1

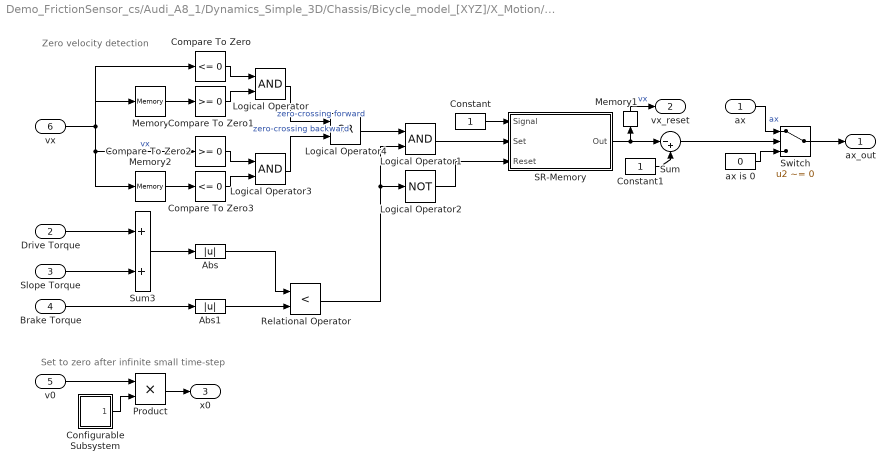
== system Demo_FrictionSensor_cs/Audi_A8_1/Dynamics_Simple_3D/Chassis/Bicycle_model_[XYZ]/X_Motion/Max RPM and zero- velocity detection ==
  note: Set to zero after infinite small time-step
  note: Zero velocity detection
  ax : Inport
  Drive Torque : Inport  Port=2
  Slope Torque : Inport  Port=3
  Brake Torque : Inport  Port=4
  v0 : Inport  Port=5
  vx : Inport  Port=6
  Abs : Abs
  Abs1 : Abs
  Compare To Zero : simulink/Logic and Bit Operations/Compare To Zero  SystemSampleTime=-1  relop=<=  LogicOutDataTypeMode=boolean  ZeroCross=off
  Compare To Zero1 : simulink/Logic and Bit Operations/Compare To Zero  SystemSampleTime=-1  relop=>=  LogicOutDataTypeMode=boolean  ZeroCross=off
  Compare To Zero2 : simulink/Logic and Bit Operations/Compare To Zero  SystemSampleTime=-1  relop=>=  LogicOutDataTypeMode=boolean  ZeroCross=off
  Compare To Zero3 : simulink/Logic and Bit Operations/Compare To Zero  SystemSampleTime=-1  relop=<=  LogicOutDataTypeMode=boolean  ZeroCross=off
  Configurable Subsystem : Subsystem  BlockChoice=Discrete Step  mask{ComputationMode=ComputationMode}
      mask prompts: ComputationMode "Compuation mode:"
      mask init:
      | SetComputationMode(gcb,ComputationMode);
      settings: AttributesFormatString=%<BlockChoice>  OpenFcn=BringToFront(gcb);  MemberBlocks=Discrete Step,Step
      settings: TemplateBlock=|
      | PreScanSimulinkLibrary/Configurable Subsystems/Step Function/Configurable
      | Subsystem
  Constant : Constant
  Constant1 : Constant
  Logical Operator : Logic  AllPortsSameDT=off  OutDataTypeStr=boolean
  Logical Operator1 : Logic  AllPortsSameDT=off  OutDataTypeStr=boolean
  Logical Operator2 : Logic  Operator=NOT  AllPortsSameDT=off  OutDataTypeStr=boolean
  Logical Operator3 : Logic  AllPortsSameDT=off  OutDataTypeStr=boolean
  Logical Operator4 : Logic  Operator=OR  AllPortsSameDT=off  OutDataTypeStr=boolean
  Memory : Memory
  Memory1 : Memory
  Memory2 : Memory
  Product : Product  RndMeth=Zero
  Relational Operator : RelationalOperator  Operator=<  OutDataTypeStr=boolean
  SR-Memory : Subsystem
  Sum : Sum  Inputs=|-+
  Sum3 : Sum  SaturateOnIntegerOverflow=on  InputSameDT=on  OutDataTypeStr=Inherit: Same as first input
  Switch : Switch  Criteria=u2 ~= 0  Threshold=0.5
  ax is 0 : Constant  Value=0
  ax_out : Outport
  vx_reset : Outport  Port=2
  x0 : Outport  Port=3
  wires:
  Logical Operator4/1 -> Logical Operator1/1
  vx/1 -> Compare To Zero/1, Compare To Zero2/1, Memory2/1, Memory/1  "vx"
  Memory2/1 -> Compare To Zero3/1
  Compare To Zero2/1 -> Logical Operator3/1
  Compare To Zero3/1 -> Logical Operator3/2
  Logical Operator3/1 -> Logical Operator4/2  "zero-crossing backward"
  Memory/1 -> Compare To Zero1/1
  Compare To Zero/1 -> Logical Operator/1
  Compare To Zero1/1 -> Logical Operator/2
  Logical Operator/1 -> Logical Operator4/1  "zero-crossing forward"
  Abs1/1 -> Relational Operator/2
  Brake Torque/1 -> Abs1/1
  Relational Operator/1 -> Logical Operator1/2, Logical Operator2/1
  Logical Operator1/1 -> SR-Memory/2(Set)
  Constant/1 -> SR-Memory/1(Signal)
  Logical Operator2/1 -> SR-Memory/3(Reset)
  SR-Memory/1(Out) -> Sum/1, Memory1/1
  Switch/1 -> ax_out/1
  Sum/1 -> Switch/2
  ax is 0/1 -> Switch/3
  Constant1/1 -> Sum/2
  v0/1 -> Product/1
  Product/1 -> x0/1
  Configurable Subsystem/1(Out1) -> Product/2
  ax/1 -> Switch/1  "ax"
  Memory1/1 -> vx_reset/1  "vx"
  Slope Torque/1 -> Sum3/2
  Drive Torque/1 -> Sum3/1
  Sum3/1 -> Abs/1
  Abs/1 -> Relational Operator/1

== system Demo_FrictionSensor_cs/Audi_A8_1/Dynamics_Simple_3D/Chassis/Bicycle_model_[XYZ]/X_Motion/No contact rear wheels ==
  ForceIn [N] : Inport
  Compare To Zero : simulink/Logic and Bit Operations/Compare To Zero  SystemSampleTime=-1  relop=~=  LogicOutDataTypeMode=boolean  ZeroCross=off
  Compare To Zero1 : simulink/Logic and Bit Operations/Compare To Zero  SystemSampleTime=-1  relop=~=  LogicOutDataTypeMode=boolean  ZeroCross=off
  Constant : Constant  Value=0
  Logical Operator : Logic  AllPortsSameDT=off  OutDataTypeStr=boolean
  Switch : Switch  Criteria=u2 ~= 0
  ForceOut [N] : Outport
  wires:
  Constant/1 -> Switch/3
  [penetrationrearleft] -> Compare To Zero/1
  [penetrationrearright] -> Compare To Zero1/1
  Compare To Zero/1 -> Logical Operator/1
  Compare To Zero1/1 -> Logical Operator/2
  Logical Operator/1 -> Switch/2
  ForceIn [N]/1 -> Switch/1
  Switch/1 -> ForceOut [N]/1

== system Demo_FrictionSensor_cs/Audi_A8_1/Dynamics_Simple_3D/Chassis/Bicycle_model_[XYZ]/X_Motion/No contact wheels ==
  ForceIn [N] : Inport
  Brake repartition : Fcn  Expr=u(1) * (u(2)/4)
  Compare To Zero{,1..3} (4 alike) : simulink/Logic and Bit Operations/Compare To Zero  SystemSampleTime=-1  relop=~=  LogicOutDataTypeMode=boolean  ZeroCross=off
  Mux : Mux  Inputs=[1 1 ]
  Sum : Sum  Inputs=++++  OutDataTypeStr=double
  ForceOut [N] : Outport
  wires:
  [penetrationrearleft] -> Compare To Zero/1
  [penetrationrearright] -> Compare To Zero1/1
  Sum/1 -> Mux/2
  ForceIn [N]/1 -> Mux/1
  [penetrationfrontleft] -> Compare To Zero2/1
  [penetrationfrontright] -> Compare To Zero3/1
  Compare To Zero2/1 -> Sum/1
  Compare To Zero3/1 -> Sum/2
  Compare To Zero/1 -> Sum/3
  Compare To Zero1/1 -> Sum/4
  Mux/1 -> Brake repartition/1
  Brake repartition/1 -> ForceOut [N]/1

== system Demo_FrictionSensor_cs/Audi_A8_1/Dynamics_Simple_3D/Chassis/Bicycle_model_[XYZ]/X_Motion/Slope Force ==
  slope_[rad] : Inport
  Fcn5 : Fcn  Expr=p.m*p.g*sin(u(1))
  SlopeForce_[N] : Outport
  wires:
  slope_[rad]/1 -> Fcn5/1  "slope_[rad]"
  Fcn5/1 -> SlopeForce_[N]/1  "SlopeForce_[N]"

== system Demo_FrictionSensor_cs/Audi_A8_1/Dynamics_Simple_3D/Chassis/Bicycle_model_[XYZ]/Y & Yaw_Motion/Configurable Subsystem ==
  In1 : Inport
  In2 : Inport  Port=2
  Discrete-Time Integrator : DiscreteIntegrator  ExternalReset=level  SampleTime=TimeStep  ICPrevOutput=DiscIntNeverNeededParam  ICPrevScaledInput=DiscIntNeverNeededParam
  Out1 : Outport
  wires:
  Discrete-Time Integrator/1 -> Out1/1
  In2/1 -> Discrete-Time Integrator/2
  In1/1 -> Discrete-Time Integrator/1

== system Demo_FrictionSensor_cs/Audi_A8_1/Dynamics_Simple_3D/Chassis/Bicycle_model_[XYZ]/Y & Yaw_Motion/Configurable Subsystem1 ==
  In1 : Inport
  In2 : Inport  Port=2
  Discrete-Time Integrator : DiscreteIntegrator  ExternalReset=level  SampleTime=TimeStep  ICPrevOutput=DiscIntNeverNeededParam  ICPrevScaledInput=DiscIntNeverNeededParam
  Out1 : Outport
  wires:
  Discrete-Time Integrator/1 -> Out1/1
  In2/1 -> Discrete-Time Integrator/2
  In1/1 -> Discrete-Time Integrator/1

== system Demo_FrictionSensor_cs/Audi_A8_1/Dynamics_Simple_3D/Chassis/Bicycle_model_[XYZ]/Y & Yaw_Motion/Configurable Subsystem2 ==
  In1 : Inport
  Discrete-Time Integrator : DiscreteIntegrator  IntegratorMethod=Integration: Backward Euler  SampleTime=TimeStep  ICPrevOutput=DiscIntNeverNeededParam  ICPrevScaledInput=DiscIntNeverNeededParam
  Out1 : Outport
  wires:
  Discrete-Time Integrator/1 -> Out1/1
  In1/1 -> Discrete-Time Integrator/1

== system Demo_FrictionSensor_cs/Audi_A8_1/Dynamics_Simple_3D/Chassis/Bicycle_model_[XYZ]/Z, Pitch_Motion & Roll_Motion/Configurable Subsystem ==
  In1 : Inport
  Discrete-Time Integrator : DiscreteIntegrator  SampleTime=TimeStep  LimitOutput=on  UpperSaturationLimit=25*pi/180  LowerSaturationLimit=-25*pi/180  ICPrevOutput=DiscIntNeverNeededParam  ICPrevScaledInput=DiscIntNeverNeededParam
  Out1 : Outport
  wires:
  Discrete-Time Integrator/1 -> Out1/1
  In1/1 -> Discrete-Time Integrator/1

== system Demo_FrictionSensor_cs/Audi_A8_1/Dynamics_Simple_3D/Chassis/Bicycle_model_[XYZ]/Z, Pitch_Motion & Roll_Motion/Configurable Subsystem1 ==
  In1 : Inport
  Discrete-Time Integrator : DiscreteIntegrator  SampleTime=TimeStep  ICPrevOutput=DiscIntNeverNeededParam  ICPrevScaledInput=DiscIntNeverNeededParam
  Out1 : Outport
  wires:
  Discrete-Time Integrator/1 -> Out1/1
  In1/1 -> Discrete-Time Integrator/1

== system Demo_FrictionSensor_cs/Audi_A8_1/Dynamics_Simple_3D/Chassis/Bicycle_model_[XYZ]/Z, Pitch_Motion & Roll_Motion/Configurable Subsystem2 ==
  In1 : Inport
  Discrete-Time Integrator : DiscreteIntegrator  SampleTime=TimeStep  ICPrevOutput=DiscIntNeverNeededParam  ICPrevScaledInput=DiscIntNeverNeededParam
  Out1 : Outport
  wires:
  Discrete-Time Integrator/1 -> Out1/1
  In1/1 -> Discrete-Time Integrator/1

== system Demo_FrictionSensor_cs/Audi_A8_1/Dynamics_Simple_3D/Chassis/Bicycle_model_[XYZ]/Z, Pitch_Motion & Roll_Motion/Configurable Subsystem3 ==
  In1 : Inport
  Discrete-Time Integrator : DiscreteIntegrator  SampleTime=TimeStep  ICPrevOutput=DiscIntNeverNeededParam  ICPrevScaledInput=DiscIntNeverNeededParam
  Out1 : Outport
  wires:
  Discrete-Time Integrator/1 -> Out1/1
  In1/1 -> Discrete-Time Integrator/1

== system Demo_FrictionSensor_cs/Audi_A8_1/Dynamics_Simple_3D/Chassis/Bicycle_model_[XYZ]/Z, Pitch_Motion & Roll_Motion/Configurable Subsystem4 ==
  In1 : Inport
  Discrete-Time Integrator : DiscreteIntegrator  SampleTime=TimeStep  ICPrevOutput=DiscIntNeverNeededParam  ICPrevScaledInput=DiscIntNeverNeededParam
  Out1 : Outport
  wires:
  Discrete-Time Integrator/1 -> Out1/1
  In1/1 -> Discrete-Time Integrator/1

== system Demo_FrictionSensor_cs/Audi_A8_1/Dynamics_Simple_3D/Chassis/Bicycle_model_[XYZ]/Z, Pitch_Motion & Roll_Motion/Configurable Subsystem5 ==
  In1 : Inport
  Discrete Derivative : PreScanSimulinkLibrary/Configurable Subsystems/Derivative/Discrete Derivative  SystemSampleTime=-1
  Out1 : Outport
  wires:
  Discrete Derivative/1 -> Out1/1
  In1/1 -> Discrete Derivative/1

== system Demo_FrictionSensor_cs/Audi_A8_1/Dynamics_Simple_3D/Chassis/Bicycle_model_[XYZ]/Z, Pitch_Motion & Roll_Motion/Configurable Subsystem6 ==
  In1 : Inport
  Discrete Derivative : PreScanSimulinkLibrary/Configurable Subsystems/Derivative/Discrete Derivative  SystemSampleTime=-1
  Out1 : Outport
  wires:
  Discrete Derivative/1 -> Out1/1
  In1/1 -> Discrete Derivative/1

== system Demo_FrictionSensor_cs/Audi_A8_1/Dynamics_Simple_3D/Chassis/Bicycle_model_[XYZ]/Z, Pitch_Motion & Roll_Motion/Configurable Subsystem7 ==
  In1 : Inport
  Discrete Derivative : PreScanSimulinkLibrary/Configurable Subsystems/Derivative/Discrete Derivative  SystemSampleTime=-1
  Out1 : Outport
  wires:
  Discrete Derivative/1 -> Out1/1
  In1/1 -> Discrete Derivative/1

== system Demo_FrictionSensor_cs/Audi_A8_1/Dynamics_Simple_3D/Chassis/Bicycle_model_[XYZ]/Z, Pitch_Motion & Roll_Motion/Configurable Subsystem8 ==
  In1 : Inport
  Discrete Derivative : PreScanSimulinkLibrary/Configurable Subsystems/Derivative/Discrete Derivative  SystemSampleTime=-1
  Out1 : Outport
  wires:
  Discrete Derivative/1 -> Out1/1
  In1/1 -> Discrete Derivative/1

== system Demo_FrictionSensor_cs/Audi_A8_1/Dynamics_Simple_3D/Chassis/Bicycle_model_[XYZ]/Z, Pitch_Motion & Roll_Motion/Configurable Subsystem9 ==
  In1 : Inport
  Discrete Derivative : PreScanSimulinkLibrary/Configurable Subsystems/Derivative/Discrete Derivative  SystemSampleTime=-1
  Out1 : Outport
  wires:
  Discrete Derivative/1 -> Out1/1
  In1/1 -> Discrete Derivative/1

== system Demo_FrictionSensor_cs/Audi_A8_1/Dynamics_Simple_3D/Chassis/Bicycle_model_[XYZ]/Z_Motion  unsprung mass/Configurable Subsystem ==
  In1 : Inport
  Derivative : Derivative
  Out1 : Outport
  wires:
  Derivative/1 -> Out1/1
  In1/1 -> Derivative/1

== system Demo_FrictionSensor_cs/Audi_A8_1/Dynamics_Simple_3D/Chassis/Bicycle_model_[XYZ]/Z_Motion  unsprung mass/Configurable Subsystem1 ==
  In1 : Inport
  Integrator : Integrator
  Out1 : Outport
  wires:
  Integrator/1 -> Out1/1
  In1/1 -> Integrator/1

== system Demo_FrictionSensor_cs/Audi_A8_1/Dynamics_Simple_3D/Chassis/Bicycle_model_[XYZ]/Z_Motion  unsprung mass/Configurable Subsystem10 ==
  In1 : Inport
  Derivative : Derivative
  Out1 : Outport
  wires:
  Derivative/1 -> Out1/1
  In1/1 -> Derivative/1

== system Demo_FrictionSensor_cs/Audi_A8_1/Dynamics_Simple_3D/Chassis/Bicycle_model_[XYZ]/Z_Motion  unsprung mass/Configurable Subsystem11 ==
  In1 : Inport
  Derivative : Derivative
  Out1 : Outport
  wires:
  Derivative/1 -> Out1/1
  In1/1 -> Derivative/1

== system Demo_FrictionSensor_cs/Audi_A8_1/Dynamics_Simple_3D/Chassis/Bicycle_model_[XYZ]/Z_Motion  unsprung mass/Configurable Subsystem2 ==
  In1 : Inport
  Integrator : Integrator
  Out1 : Outport
  wires:
  Integrator/1 -> Out1/1
  In1/1 -> Integrator/1

== system Demo_FrictionSensor_cs/Audi_A8_1/Dynamics_Simple_3D/Chassis/Bicycle_model_[XYZ]/Z_Motion  unsprung mass/Configurable Subsystem3 ==
  In1 : Inport
  Integrator : Integrator
  Out1 : Outport
  wires:
  Integrator/1 -> Out1/1
  In1/1 -> Integrator/1

== system Demo_FrictionSensor_cs/Audi_A8_1/Dynamics_Simple_3D/Chassis/Bicycle_model_[XYZ]/Z_Motion  unsprung mass/Configurable Subsystem4 ==
  In1 : Inport
  Integrator : Integrator
  Out1 : Outport
  wires:
  Integrator/1 -> Out1/1
  In1/1 -> Integrator/1

== system Demo_FrictionSensor_cs/Audi_A8_1/Dynamics_Simple_3D/Chassis/Bicycle_model_[XYZ]/Z_Motion  unsprung mass/Configurable Subsystem5 ==
  In1 : Inport
  Integrator : Integrator
  Out1 : Outport
  wires:
  Integrator/1 -> Out1/1
  In1/1 -> Integrator/1

== system Demo_FrictionSensor_cs/Audi_A8_1/Dynamics_Simple_3D/Chassis/Bicycle_model_[XYZ]/Z_Motion  unsprung mass/Configurable Subsystem6 ==
  In1 : Inport
  Integrator : Integrator
  Out1 : Outport
  wires:
  Integrator/1 -> Out1/1
  In1/1 -> Integrator/1

== system Demo_FrictionSensor_cs/Audi_A8_1/Dynamics_Simple_3D/Chassis/Bicycle_model_[XYZ]/Z_Motion  unsprung mass/Configurable Subsystem7 ==
  In1 : Inport
  Integrator : Integrator
  Out1 : Outport
  wires:
  Integrator/1 -> Out1/1
  In1/1 -> Integrator/1

== system Demo_FrictionSensor_cs/Audi_A8_1/Dynamics_Simple_3D/Chassis/Bicycle_model_[XYZ]/Z_Motion  unsprung mass/Configurable Subsystem8 ==
  In1 : Inport
  Integrator : Integrator
  Out1 : Outport
  wires:
  Integrator/1 -> Out1/1
  In1/1 -> Integrator/1

== system Demo_FrictionSensor_cs/Audi_A8_1/Dynamics_Simple_3D/Chassis/Bicycle_model_[XYZ]/Z_Motion  unsprung mass/Configurable Subsystem9 ==
  In1 : Inport
  Derivative : Derivative
  Out1 : Outport
  wires:
  Derivative/1 -> Out1/1
  In1/1 -> Derivative/1

== system Demo_FrictionSensor_cs/Audi_A8_1/Dynamics_Simple_3D/Chassis/FrontTyre/AlphaFront/Enabled Subsystem ==
  In : Inport
  Enable : EnablePort  PropagateVarSize=During execution
  AlphaFront : Fcn  Expr=-atan( (u(2)+u(3)*p.a)/u(1) )
  Alpha : Outport  OutputWhenDisabled=reset  InitialOutput=[0]
  wires:
  In/1 -> AlphaFront/1
  AlphaFront/1 -> Alpha/1

== system Demo_FrictionSensor_cs/Audi_A8_1/Dynamics_Simple_3D/Chassis/RearTyre/AlphaRear/Enabled Subsystem ==
  In : Inport
  Enable : EnablePort  PropagateVarSize=During execution
  AlphaRear : Fcn  Expr=-atan( (u(2)-u(3)*p.b)/u(1) )
  Alpha : Outport  OutputWhenDisabled=reset  InitialOutput=[0]
  wires:
  In/1 -> AlphaRear/1
  AlphaRear/1 -> Alpha/1

== system Demo_FrictionSensor_cs/Audi_A8_1/PreScan_Contact_Sensor/Vehicle Local to World/state2FullState/limit roll/Substitute 90 & 270 deg (and its plurals) ==
  Angle [rad] : Inport
  270 deg detection : simulink/Model Verification/Check  Static Gap  Description=u <= 269.5 || 270.5 <= u  SystemSampleTime=-1  max=270.5  max_included=on  min=269.5  min_included=on  enabled=on  stopWhenAssertionFail=off  export=on  icon=graphic
  90 deg detection : simulink/Model Verification/Check  Static Gap  Description=u <= 89.5 || 90.5 <= u  SystemSampleTime=-1  max=90.5  max_included=on  min=89.5  min_included=on  enabled=on  stopWhenAssertionFail=off  export=on  icon=graphic
  Angle 0-360 deg limiter : Subsystem
  Degrees to Radians : simulink_extras/Transformations/Degrees to Radians  SystemSampleTime=-1
  Radians to Degrees : simulink_extras/Transformations/Radians to Degrees  SystemSampleTime=-1
  Substitution  Value : Constant  Value=269.5
  Substitution Value : Constant  Value=89.5
  Switch : Switch  Threshold=0.5
  Switch1 : Switch  Threshold=0.5
  Subst Angle [rad] : Outport
  wires:
  Angle 0-360 deg limiter/1(LimAngle [deg]) -> Switch/1, 90 deg detection/1
  90 deg detection/1 -> Switch/2
  Substitution Value/1 -> Switch/3
  Switch/1 -> 270 deg detection/1, Switch1/1
  270 deg detection/1 -> Switch1/2
  Substitution  Value/1 -> Switch1/3
  Switch1/1 -> Degrees to Radians/1
  Radians to Degrees/1 -> Angle 0-360 deg limiter/1(Angle [deg])
  Degrees to Radians/1 -> Subst Angle [rad]/1
  Angle [rad]/1 -> Radians to Degrees/1

== system Demo_FrictionSensor_cs/Audi_A8_1/Trajectories/Traj2State1/Traj2State2/Traj2MuxState_Ext/demux ==
  traj : Inport
  Demux : Demux  Outputs=18
  x : Outport
  y : Outport  Port=2
  z : Outport  Port=3
  velx : Outport  Port=4
  vely : Outport  Port=5
  velz : Outport  Port=6
  R : Outport  Port=7
  P : Outport  Port=8
  Y : Outport  Port=9
  velR : Outport  Port=10
  velP : Outport  Port=11
  velY : Outport  Port=12
  accx : Outport  Port=13
  accy : Outport  Port=14
  accz : Outport  Port=15
  accR : Outport  Port=16
  accP : Outport  Port=17
  accY : Outport  Port=18
  wires:
  Demux/18 -> accY/1
  Demux/17 -> accP/1
  Demux/16 -> accR/1
  Demux/15 -> accz/1
  Demux/14 -> accy/1
  Demux/13 -> accx/1
  Demux/12 -> velY/1
  Demux/11 -> velP/1
  Demux/10 -> velR/1
  Demux/9 -> velz/1
  Demux/8 -> vely/1
  Demux/7 -> velx/1
  Demux/6 -> Y/1
  Demux/5 -> P/1
  traj/1 -> Demux/1
  Demux/4 -> R/1
  Demux/3 -> z/1
  Demux/2 -> y/1
  Demux/1 -> x/1

== system Demo_FrictionSensor_cs/Audi_A8_1/Dynamics_Simple_3D/Chassis/Bicycle_model_[XYZ]/RoadContact/RoadGeometry/Calc_banking ==
  zi : Inport
  Constant : Constant  Value=[1, -1, 1, -1]
  Gain : Gain  Gain=1/(p.width*2)
  Product : Product  RndMeth=Zero
  Saturation : Saturate  UpperLimit=1  LowerLimit=-1
  Sum of Elements : Sum  Inputs=+
  Trigonometric Function : Trigonometry  Operator=asin
  banking : Outport
  wires:
  Trigonometric Function/1 -> banking/1
  Sum of Elements/1 -> Gain/1
  Gain/1 -> Saturation/1
  Product/1 -> Sum of Elements/1
  Constant/1 -> Product/2
  zi/1 -> Product/1
  Saturation/1 -> Trigonometric Function/1

== system Demo_FrictionSensor_cs/Audi_A8_1/Dynamics_Simple_3D/Chassis/Bicycle_model_[XYZ]/RoadContact/RoadGeometry/Calc_slope ==
  zi : Inport
  Constant : Constant  Value=[-1, -1, 1, 1]
  Gain : Gain  Gain=1/(p.l*2)
  Product : Product  RndMeth=Zero
  Saturation : Saturate  UpperLimit=1  LowerLimit=-1
  Sum of Elements : Sum  Inputs=+
  Trigonometric Function : Trigonometry  Operator=asin
  slope : Outport
  wires:
  Trigonometric Function/1 -> slope/1
  Sum of Elements/1 -> Gain/1
  Gain/1 -> Saturation/1
  Product/1 -> Sum of Elements/1
  Constant/1 -> Product/2
  zi/1 -> Product/1
  Saturation/1 -> Trigonometric Function/1

== system Demo_FrictionSensor_cs/Audi_A8_1/Dynamics_Simple_3D/Chassis/Bicycle_model_[XYZ]/RoadContact/RoadGeometry/Calc_z ==
  zi : Inport
  zC : Subsystem
  z : Outport
  wires:
  zi/1 -> zC/1(Array)
  zC/1(Mean) -> z/1

== system Demo_FrictionSensor_cs/Audi_A8_1/Dynamics_Simple_3D/Chassis/Bicycle_model_[XYZ]/RoadContact/RoadGeometry/zFL_lowerpenetrationdetph ==
  penetrationdepth : Inport
  position_z : Inport  Port=2
  normal_z : Inport  Port=3
  Add : Sum  Inputs=-+
  Configurable Subsystem : Subsystem  BlockChoice=Discrete Transfer Fcn  mask{ComputationMode=ComputationMode}
      mask prompts: ComputationMode "Compuation mode:"
      mask init:
      | SetComputationMode(gcb,ComputationMode);
      settings: AttributesFormatString=%<BlockChoice>  OpenFcn=BringToFront(gcb);  MemberBlocks=Discrete Transfer Fcn,Transfer Fcn
      settings: TemplateBlock=|
      | PreScanSimulinkLibrary/Configurable Subsystems/TransferFunction
      | lowerpenetrationdetph/Configurable
      | Subsystem
  Constant : Constant  Value=Inf
  Constant1 : Constant  Value=-6
  Constant2 : Constant  Value=-Inf
  MinMax : MinMax
  Product : Product  RndMeth=Zero
  Product1 : Product  Inputs=/*  RndMeth=Zero
  Product2 : Product  RndMeth=Zero
  Rate Limiter Dynamic : simulink/Discontinuities/Rate Limiter Dynamic  SystemSampleTime=-1
  Relational Operator : RelationalOperator  Operator===  OutDataTypeStr=boolean
  Sum of Elements : Sum  Inputs=+
  Sum of Elements1 : Sum  Inputs=+
  Sum of Elements2 : Sum  Inputs=+
  Switch : Switch
  z : Outport
  wires:
  Configurable Subsystem/1(Out1) -> z/1
  Rate Limiter Dynamic/1 -> Configurable Subsystem/1(In1)
  Switch/1 -> Rate Limiter Dynamic/3
  Constant2/1 -> Switch/3
  Constant1/1 -> Switch/1
  Sum of Elements2/1 -> Switch/2
  Constant/1 -> Rate Limiter Dynamic/1
  Product1/1 -> Rate Limiter Dynamic/2
  position_z/1 -> Add/2
  Product2/1 -> Add/1
  Sum of Elements/1 -> Product1/2
  Sum of Elements1/1 -> Product1/1
  Relational Operator/1 -> Sum of Elements1/1, Product/1
  Product/1 -> Sum of Elements/1
  MinMax/1 -> Relational Operator/2
  penetrationdepth/1 -> Sum of Elements2/1, Relational Operator/1, MinMax/1, Product2/1
  Add/1 -> Product/2
  normal_z/1 -> Product2/2

== system Demo_FrictionSensor_cs/Audi_A8_1/Dynamics_Simple_3D/Chassis/Bicycle_model_[XYZ]/RoadContact/RoadGeometry/zFL_tyreinfo ==
  In1 : Inport
  Bus Selector2 : BusSelector  OutputSignals=TireFL.cp0.penetrationdepth,TireFL.cp1.penetrationdepth,TireFL.cp2.penetrationdepth,TireFL.cp3.penetrationdepth,TireFL.cp0.position.z,TireFL.cp1.position.z,TireFL.cp2.position.z,TireFL.cp3.position.z,TireFL.cp0.normal.z,TireFL.cp1.normal.z,TireFL.cp2.normal.z,TireFL.cp3.normal.z
  Mux11 : Mux
  Mux12 : Mux
  Mux13 : Mux
  penetrationdepth : Outport
  position_z : Outport  Port=2
  normal_z : Outport  Port=3
  wires:
  Mux13/1 -> normal_z/1
  Mux12/1 -> position_z/1
  Mux11/1 -> penetrationdepth/1
  In1/1 -> Bus Selector2/1
  Bus Selector2/12 -> Mux13/4  "<z>"
  Bus Selector2/11 -> Mux13/3  "<z>"
  Bus Selector2/10 -> Mux13/2  "<z>"
  Bus Selector2/9 -> Mux13/1  "<z>"
  Bus Selector2/8 -> Mux12/4  "<z>"
  Bus Selector2/7 -> Mux12/3  "<z>"
  Bus Selector2/6 -> Mux12/2  "<z>"
  Bus Selector2/5 -> Mux12/1  "<z>"
  Bus Selector2/4 -> Mux11/4  "<penetrationdepth>"
  Bus Selector2/3 -> Mux11/3  "<penetrationdepth>"
  Bus Selector2/2 -> Mux11/2  "<penetrationdepth>"
  Bus Selector2/1 -> Mux11/1  "<penetrationdepth>"

== system Demo_FrictionSensor_cs/Audi_A8_1/Dynamics_Simple_3D/Chassis/Bicycle_model_[XYZ]/RoadContact/RoadGeometry/zFR_lowerpenetrationdetph ==
  penetrationdepth : Inport
  position_z : Inport  Port=2
  normal_z : Inport  Port=3
  Add : Sum  Inputs=-+
  Configurable Subsystem : Subsystem  BlockChoice=Discrete Transfer Fcn  mask{ComputationMode=ComputationMode}
      mask prompts: ComputationMode "Compuation mode:"
      mask init:
      | SetComputationMode(gcb,ComputationMode);
      settings: AttributesFormatString=%<BlockChoice>  OpenFcn=BringToFront(gcb);  MemberBlocks=Discrete Transfer Fcn,Transfer Fcn
      settings: TemplateBlock=|
      | PreScanSimulinkLibrary/Configurable Subsystems/TransferFunction
      | lowerpenetrationdetph/Configurable
      | Subsystem
  Constant : Constant  Value=Inf
  Constant1 : Constant  Value=-6
  Constant2 : Constant  Value=-Inf
  MinMax : MinMax
  Product : Product  RndMeth=Zero
  Product1 : Product  Inputs=/*  RndMeth=Zero
  Product2 : Product  RndMeth=Zero
  Rate Limiter Dynamic : simulink/Discontinuities/Rate Limiter Dynamic  SystemSampleTime=-1
  Relational Operator : RelationalOperator  Operator===  OutDataTypeStr=boolean
  Sum of Elements : Sum  Inputs=+
  Sum of Elements1 : Sum  Inputs=+
  Sum of Elements2 : Sum  Inputs=+
  Switch : Switch
  z : Outport
  wires:
  normal_z/1 -> Product2/2
  Add/1 -> Product/2
  penetrationdepth/1 -> Product2/1, MinMax/1, Relational Operator/1, Sum of Elements2/1
  MinMax/1 -> Relational Operator/2
  Product/1 -> Sum of Elements/1
  Relational Operator/1 -> Product/1, Sum of Elements1/1
  Sum of Elements1/1 -> Product1/1
  Sum of Elements/1 -> Product1/2
  Product2/1 -> Add/1
  position_z/1 -> Add/2
  Product1/1 -> Rate Limiter Dynamic/2
  Constant/1 -> Rate Limiter Dynamic/1
  Sum of Elements2/1 -> Switch/2
  Constant1/1 -> Switch/1
  Constant2/1 -> Switch/3
  Switch/1 -> Rate Limiter Dynamic/3
  Rate Limiter Dynamic/1 -> Configurable Subsystem/1(In1)
  Configurable Subsystem/1(Out1) -> z/1
